simulink model "Vacuum_degassifier_discontinuous"  (Simulink 8.5)
settings: Solver=ode15s  SolverMode=SingleTasking  StartTime=0.0  StopTime=2*3600  MaxStep=10  RelTol=1e-5  AbsTol=1e-5
undefined symbols (not defined in the file): B, U, x0
settings Model: Creator=psross  LastModifiedBy=Martijn  ExtModeTrigMode=oneshot  ExtModeArmWhenConnect=off
settings DataIOCC: LimitDataPoints=off  SaveOutput=off  SaveTime=off  SignalLoggingName=sigsOut
settings OptimizationCC: BooleanDataType=off
settings DebuggingCC: SaveWithParameterizedLinksMsg=none  SignalResolutionControl=TryResolveAllWithWarning  MultiTaskDSMMsg=warning  MultiTaskCondExecSysMsg=none  FcnCallInpInsideContextMsg=UseLocalSettings  StrictBusMsg=None
settings HardwareCC: TargetUnknown=on

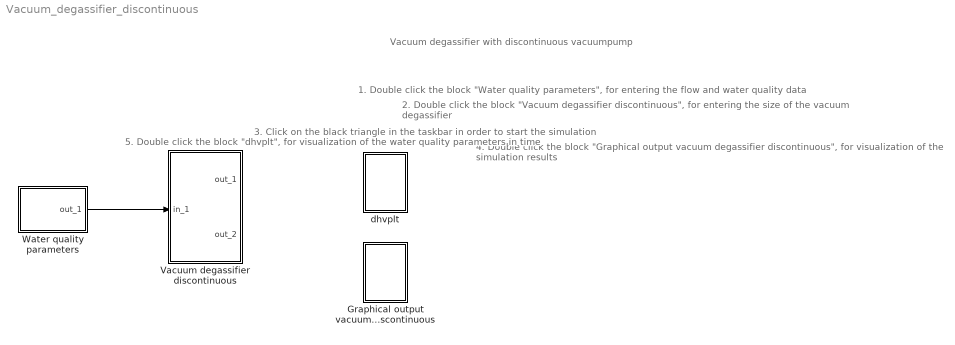
== system Vacuum_degassifier_discontinuous ==
  note: Vacuum degassifier with discontinuous vacuumpump
  note: 2. Double click the block "Vacuum degassifier discontinuous", for entering the size of the vacuum degassifier
  note: 3. Click on the black triangle in the taskbar in order to start the simulation
  note: 4. Double click the block "Graphical output vacuum degassifier discontinuous", for visualization of the simulation results
  note: 1. Double click the block "Water quality parameters", for entering the flow and water quality data
  note: 5. Double click the block "dhvplt", for visualization of the water quality parameters in time
  "Graphical output vacuum degassifier discontinuous " : Subsystem
      settings: OpenFcn=vacuum_g
      mask Display:
      | plot(0,0,100,100,[80,20,20],[20,20,80],[80,69,60,52,45,39,33,28,24,20],[65,65,64,61,57,52,45,37,30,20])
      | disp('');
      | text(100,100,'vacuum', 'horizontalAlignment', 'right', 'verticalAlignment', 'top');
  Vacuum degassifier discontinuous : Subsystem  Description=This model calculates the degassifying with a vacuum degassifier with a discontinuous vacuumpump. The influent carbon dioxide concentration is calculated on the basis of the bicarbonate concentration, the pH, the EGV and the water temperature, so these parameters must always be filled out in the 'Water quality parameters' block.
      mask init:
      | filenaam='./StimelaData/Vacuum_discontinuous.mat';
      | 
      | [Pn,Fn,Fext]=Fileprop(filenaam);
      | 
      | errstr = st_UniqName(filenaam,'filenaam=''','SubSystem','OpenFcn');
      | if errstr, error([errstr 'The filename "' filenaam '" is already in use. Choose a different filename.']), end
      | 
      | P = vacuum_p(filenaam);
      | [B,x0,U]=vacuum_i(filenaam);
      settings: OpenFcn=|
      | filenaam='./StimelaData/Vacuum_discontinuous.mat';
      | st_ParameterInput('init',gcb,filenaam,'vacuum');
      mask Display:
      | plot(0,0,100,100,[20,20],[20,80],[80,80],[20,80],[20,80,20,80,20],[30,70,70,30,30],[80,20],[28,28],[50,44,34,27,23,20],[90,90,89,87,84,80],[50,44,34,27,23,20],[10,10,11,13,16,20],[50,56,66,73,77,80],[90,90,89,87,84,80],[50,56,66,73,77,80],[10,10,11,13,16,20],[21,20],[82,80],[10,50,50,10],[82,82,80,80],[58,50,42],[76,80,76],[45,45],[3,10],[55,55],[3,10])
      | disp('')
      | text(50,50,'vacuum', 'horizontalAlignment', 'center', 'verticalAlignment', 'middle');
      | text(50,0,Fn, 'horizontalAlignment', 'center', 'verticalAlignment', 'base');
  Water quality parameters : Subsystem  Description=The water flow and the water quality data must be filled out in the 'Water quality parameters' block. Each project must start with a 'Water quality parameters' block.
      mask init:
      | filenaam='./StimelaData/Water_qual_param.mat';
      | 
      | [Pn,Fn,Fext]=Fileprop(filenaam);
      | 
      | errstr = st_UniqName(filenaam,'filenaam=''','SubSystem','OpenFcn');
      | if errstr, error([errstr 'The filename "' filenaam '" is already in use. Choose a different filename.']), end
      | 
      | P = invruw_p(filenaam);
      | [B,x0,U]=invruw_i(filenaam);
      settings: OpenFcn=|
      | filenaam='./StimelaData/Water_qual_param.mat';
      | st_ParameterInput('init',gcb,filenaam,'invruw');
      mask Display:
      | plot(0,0,100,100,[80 100],[ 50 50],[80 100],[ 55 55],[20 80 80 20 20],[10 10 90  90 10]);
      | disp('')
      | text(50,50,'invruw', 'horizontalAlignment', 'center', 'verticalAlignment', 'middle');
      | text(50,0,Fn, 'horizontalAlignment', 'center', 'verticalAlignment', 'base');
  dhvplt : Subsystem
      settings: OpenFcn=plotStimela2
      mask Display:
      | plot(0,0,100,100,[80,20,20],[20,20,80],[80,69,60,52,45,39,33,28,24,20],[65,65,64,61,57,52,45,37,30,20])
      | disp('');
      | text(100,100,'Stimela', 'horizontalAlignment', 'right', 'verticalAlignment', 'top');
  wires:
  Water quality parameters/1(out_1) -> Vacuum degassifier discontinuous/1(in_1)

== system Vacuum_degassifier_discontinuous/Graphical output vacuum degassifier discontinuous  ==
  note: plotten

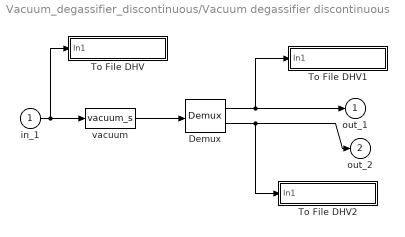
== system Vacuum_degassifier_discontinuous/Vacuum degassifier discontinuous ==
  in_1 : Inport
  Demux : Demux  Outputs=[U.Number B.Measurements]
  To File DHV : Subsystem  mask(To File DHV){naam=[filenaam(1:length(filenaam)-4) '_in.sti']}
      mask prompts: naam "Naam van bestand"
      mask init:
      | set_param([gcb '/To File'],'Filename',naam);
      mask Display: disp(naam)
  To File DHV1 : Subsystem  mask(To File DHV){naam=[filenaam(1:length(filenaam)-4) '_out.sti']}
      mask prompts: naam "Naam van bestand"
      mask init:
      | set_param([gcb '/To File'],'Filename',naam);
      mask Display: disp(naam)
  To File DHV2 : Subsystem  mask(To File DHV){naam=[filenaam(1:length(filenaam)-4) '_EM.sti']}
      mask prompts: naam "Naam van bestand"
      mask init:
      | set_param([gcb '/To File'],'Filename',naam);
      mask Display: disp(naam)
  vacuum : S-Function  FunctionName=vacuum_s  Parameters=B,x0,U,P
  out_1 : Outport  InitialOutput=0
  out_2 : Outport  Port=2  InitialOutput=0
  wires:
  vacuum/1 -> Demux/1
  Demux/1 -> out_1/1, To File DHV1/1(In1)
  Demux/2 -> out_2/1, To File DHV2/1(In1)
  in_1/1 -> vacuum/1, To File DHV/1(In1)

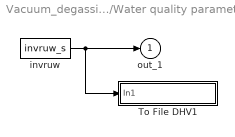
== system Vacuum_degassifier_discontinuous/Water quality parameters ==
  To File DHV1 : Subsystem  mask(To File DHV){naam=[filenaam(1:length(filenaam)-4) '_out.sti']}
      mask prompts: naam "Naam van bestand"
      mask init:
      | set_param([gcb '/To File'],'Filename',naam);
      mask Display: disp(naam)
  invruw : S-Function  FunctionName=invruw_s  Parameters=B,x0,U,P
  out_1 : Outport  InitialOutput=0
  wires:
  invruw/1 -> out_1/1, To File DHV1/1(In1)

== system Vacuum_degassifier_discontinuous/dhvplt ==
  note: plotten

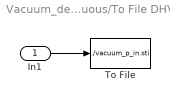
== system Vacuum_degassifier_discontinuous/Vacuum degassifier discontinuous/To File DHV ==
  In1 : Inport
  To File : ToFile  Filename=./vacuum_p_in.sti  MatrixName=vacuumin
  wires:
  In1/1 -> To File/1

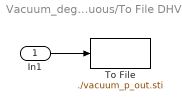
== system Vacuum_degassifier_discontinuous/Vacuum degassifier discontinuous/To File DHV1 ==
  In1 : Inport
  To File : ToFile  Filename=./vacuum_p_out.sti  MatrixName=vacuumout
  wires:
  In1/1 -> To File/1

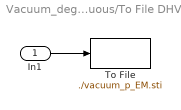
== system Vacuum_degassifier_discontinuous/Vacuum degassifier discontinuous/To File DHV2 ==
  In1 : Inport
  To File : ToFile  Filename=./vacuum_p_EM.sti  MatrixName=vacuumEM
  wires:
  In1/1 -> To File/1

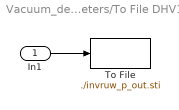
== system Vacuum_degassifier_discontinuous/Water quality parameters/To File DHV1 ==
  In1 : Inport
  To File : ToFile  Filename=./invruw_p_out.sti  MatrixName=invruwout
  wires:
  In1/1 -> To File/1
